simulink model "mixTest123"  (R2020a)
settings: Solver=VariableStepAuto  StartTime=0.0  StopTime=1000  FixedStep=0.05  RelTol=1e-3
InitFcn:
  | data_current
values from neighbouring files (symbols this model uses):
  a1 = rho * D^4 * alpha1    (= 0.000388302366464)    [data_current.m]    (also in main_init.m)
  a2 = -rho * D^3 * alpha2 * (1 - omega)    (= 0.0037030698432)    [data_current.m]    (also in main_init.m)
  ag = [Ax Ay Az]'    [init_modello.m]
  alpha1 = 0.0113    [data_current.m]    (also in main_init.m)
  alpha2 = -0.0091    [data_current.m]    (also in main_init.m)
  areaOfInterestCorner = [42.317744;10.915136; 0]    [init_controllo.m]    (also in missionA.m = [42.317744)
  bg = [Bx By Bz]'    [init_modello.m]
  cd_pitch = 0.7    [init_modello.m]
  cd_roll = 0.04    [init_modello.m]
  cd_x = 0.4    [init_modello.m]
  cd_y = 1    [init_modello.m]
  cd_yaw = 0.7    [init_modello.m]
  cd_z = 1    [init_modello.m]
  cg = [Cx Cy Cz]'    [init_modello.m]
  D = 0.076    [data_current.m]    (also in main_init.m)
  dead_zone_limit = 31.5    [data_current.m]    (also in main_init.m)
  dg = [Dx Dy Dz]'    [init_modello.m]
  eg = [Ex Ey Ez]'    [init_modello.m]
  fg = [Fx Fy Fz]'    [init_modello.m]
  g = 9.81    [init_modello.m]
  galleggiamento = 66.5386    [init_controllo.m]
  gg = [Gx Gy Gz]'    [init_modello.m]
  H0 = 0    [init_modello.m]
  init_position = [pointP(1),pointP(2),0.15,0,0,deg2rad(angle)]'    [appunti.m]    (also in init_modello.m = [pointP(1),pointP(2),0.15,0,0,deg2rad(alpha)]')
  init_velocity = [0 0 0 0 0 0]'    [init_modello.m]
  Ixx = 0.93304097392    [init_modello.m]
  Ixy = 0    [init_modello.m]
  Ixz = 0    [init_modello.m]
  Iyy = 25.58745481378    (= 25.5874548138)    [init_modello.m]
  Iyz = 0    [init_modello.m]
  Izz = 25.58745481378    (= 25.5874548138)    [init_modello.m]
  K_i_heave_div = 20    [init_controllo.m]
  K_i_heave_pos = 1    [init_controllo.m]
  K_i_heave_surf = 20    [init_controllo.m]
  K_i_heave_trans = 5    [init_controllo.m]
  K_i_heave_turn = 5    [init_controllo.m]
  K_i_pitch_div = 0    [init_controllo.m]
  K_i_pitch_pos = 0.1*0    (= 0)    [init_controllo.m]
  K_i_pitch_surf = 0    [init_controllo.m]
  K_i_pitch_trans = 0    [init_controllo.m]
  K_i_pitch_turn = 0    [init_controllo.m]
  K_i_roll_div = 0    [init_controllo.m]
  K_i_roll_pos = 0.1*0    (= 0)    [init_controllo.m]
  K_i_roll_surf = 1    [init_controllo.m]
  K_i_roll_trans = 0    [init_controllo.m]
  K_i_roll_turn = 0    [init_controllo.m]
  K_i_surge_div = 3    [init_controllo.m]
  K_i_surge_pos = 0.1679*30    (= 5.037)    [init_controllo.m]
  K_i_surge_surf = 3    [init_controllo.m]
  K_i_surge_trans = 0.1679*15    (= 2.5185)    [init_controllo.m]
  K_i_surge_turn = 0.1679*60    (= 10.074)    [init_controllo.m]
  K_i_sway_div = 6    [init_controllo.m]
  K_i_sway_pos = 5    [init_controllo.m]
  K_i_sway_surf = 3    [init_controllo.m]
  K_i_sway_trans = 2    [init_controllo.m]
  K_i_sway_turn = 50    [init_controllo.m]
  K_i_yaw_div = 0    [init_controllo.m]
  K_i_yaw_pos = 1    [init_controllo.m]
  K_i_yaw_surf = 0    [init_controllo.m]
  K_i_yaw_trans = 20    [init_controllo.m]
  K_i_yaw_turn = 3    [init_controllo.m]
  K_p_heave_div = 200    [init_controllo.m]
  K_p_heave_pos = 320    [init_controllo.m]
  K_p_heave_surf = 200    [init_controllo.m]
  K_p_heave_trans = 170    [init_controllo.m]
  K_p_heave_turn = 170    [init_controllo.m]
  K_p_phi_div = 0.15    [init_controllo.m]
  K_p_phi_pos = 1*0.1    (= 0.1)    [init_controllo.m]
  K_p_phi_surf = 0.15    [init_controllo.m]
  K_p_phi_trans = 0.1    [init_controllo.m]
  K_p_phi_turn = 0.1    [init_controllo.m]
  K_p_pitch_div = 50    [init_controllo.m]
  K_p_pitch_pos = 25    [init_controllo.m]
  K_p_pitch_surf = 50    [init_controllo.m]
  K_p_pitch_trans = 25    [init_controllo.m]
  K_p_pitch_turn = 25    [init_controllo.m]
  K_p_psi_div = 0.3    [init_controllo.m]
  K_p_psi_pos = 0.25    [init_controllo.m]
  K_p_psi_surf = 0.3    [init_controllo.m]
  K_p_psi_trans = 0.2    [init_controllo.m]
  K_p_roll_div = 10    [init_controllo.m]
  K_p_roll_pos = 0.1*40    (= 4)    [init_controllo.m]
  K_p_roll_surf = 10    [init_controllo.m]
  K_p_roll_trans = 0.1*40    (= 4)    [init_controllo.m]
  K_p_roll_turn = 4    [init_controllo.m]
  K_p_surge_div = 80    [init_controllo.m]
  K_p_surge_pos = 13.7782*2.5    (= 34.4455)    [init_controllo.m]
  K_p_surge_surf = 80    [init_controllo.m]
  K_p_surge_trans = 20    [init_controllo.m]
  K_p_surge_turn = 150    [init_controllo.m]
  K_p_sway_div = 100    [init_controllo.m]
  K_p_sway_pos = 90    [init_controllo.m]
  K_p_sway_surf = 80    [init_controllo.m]
  K_p_sway_trans = 80    [init_controllo.m]
  K_p_sway_turn = 200    [init_controllo.m]
  K_p_th_div = 0.3    [init_controllo.m]
  K_p_th_pos = 0.1    [init_controllo.m]
  K_p_th_surf = 0.3    [init_controllo.m]
  K_p_th_trans = 0.1    [init_controllo.m]
  K_p_th_turn = 0.1    [init_controllo.m]
  K_p_x_div = 0.12    [init_controllo.m]
  K_p_x_pos = 0.12    [init_controllo.m]
  K_p_x_surf = 0.12    [init_controllo.m]
  K_p_y_div = 0.6    [init_controllo.m]
  K_p_y_pos = 0.34    [init_controllo.m]
  K_p_y_surf = 0.1    [init_controllo.m]
  K_p_y_trans = 0.3    [init_controllo.m]
  K_p_y_turn = 0.3    [init_controllo.m]
  K_p_yaw_div = 70    [init_controllo.m]
  K_p_yaw_pos = 20    [init_controllo.m]
  K_p_yaw_surf = 70    [init_controllo.m]
  K_p_yaw_trans = 160    [init_controllo.m]
  K_p_yaw_turn = 60    [init_controllo.m]
  K_p_z_div = 0.35    [init_controllo.m]
  K_p_z_pos = 0.2    [init_controllo.m]
  K_p_z_surf = 0.35    [init_controllo.m]
  K_p_z_trans = 0.10    (= 0.1)    [init_controllo.m]
  K_p_z_turn = 0.1    [init_controllo.m]
  Kadd = 0    [init_modello.m]
  m = 100    [init_modello.m]    (also in retta.m = p2-p1)
  ... (+29 more)
undefined symbols (not defined in the file or in its folder): DiscIntNeverNeededParam
libraries: simulink x4
(part 3 of 5)

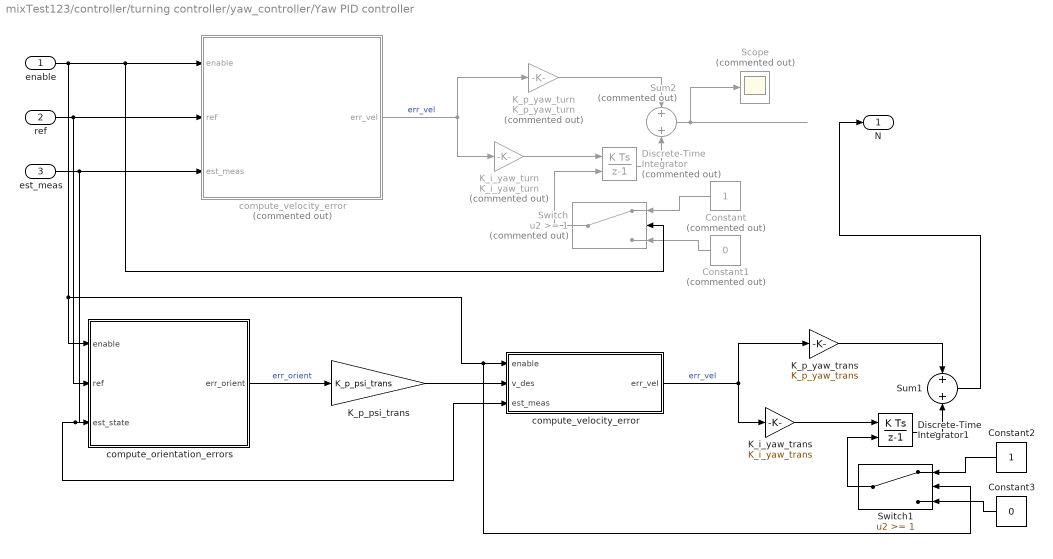
== system mixTest123/controller/turning controller/yaw_controller/Yaw PID controller ==
  enable : Inport
  ref : Inport  Port=2
  est_meas : Inport  Port=3
  " compute_velocity_error" : MATLAB Function  Commented=on  TreatAsAtomicUnit=on
  Constant : Constant  Commented=on
  Constant1 : Constant  Commented=on  Value=0
  Constant2 : Constant
  Constant3 : Constant  Value=0
  Discrete-Time Integrator : DiscreteIntegrator  Commented=on  ExternalReset=falling  SampleTime=0.1  ICPrevOutput=DiscIntNeverNeededParam  ICPrevScaledInput=DiscIntNeverNeededParam
  Discrete-Time Integrator1 : DiscreteIntegrator  ExternalReset=falling  SampleTime=0.1  ICPrevOutput=DiscIntNeverNeededParam  ICPrevScaledInput=DiscIntNeverNeededParam
  K_i_yaw_trans : Gain  Gain=K_i_yaw_trans
  K_i_yaw_turn : Gain  Commented=on  Gain=K_i_yaw_turn
  K_p_psi_trans : Gain  Gain=K_p_psi_trans
  K_p_yaw_trans : Gain  Gain=K_p_yaw_trans
  K_p_yaw_turn : Gain  Commented=on  Gain=K_p_yaw_turn
  Scope : Scope  Commented=on
  Sum1 : Sum
  Sum2 : Sum  Commented=on
  Switch : Switch  Commented=on  Threshold=1
  Switch1 : Switch  Threshold=1
  compute_orientation_errors : MATLAB Function  TreatAsAtomicUnit=on
  compute_velocity_error : MATLAB Function  TreatAsAtomicUnit=on
  N : Outport
  wires:
  Sum2/1 -> Scope/1
  " compute_velocity_error"/1(err_vel) -> K_i_yaw_turn/1, K_p_yaw_turn/1  "err_vel"
  Discrete-Time Integrator/1 -> Sum2/2
  K_p_yaw_turn/1 -> Sum2/1
  K_i_yaw_turn/1 -> Discrete-Time Integrator/1
  Switch/1 -> Discrete-Time Integrator/2
  Constant1/1 -> Switch/3
  Constant/1 -> Switch/1
  Constant3/1 -> Switch1/3
  Constant2/1 -> Switch1/1
  K_p_psi_trans/1 -> compute_velocity_error/2(v_des)
  Switch1/1 -> Discrete-Time Integrator1/2
  compute_velocity_error/1(err_vel) -> K_i_yaw_trans/1, K_p_yaw_trans/1  "err_vel"
  enable/1 -> compute_orientation_errors/1(enable), Switch1/2, compute_velocity_error/1(enable), Switch/2, " compute_velocity_error"/1(enable)
  K_i_yaw_trans/1 -> Discrete-Time Integrator1/1
  compute_orientation_errors/1(err_orient) -> K_p_psi_trans/1  "err_orient"
  est_meas/1 -> " compute_velocity_error"/3(est_meas), compute_velocity_error/3(est_meas), compute_orientation_errors/3(est_state)
  K_p_yaw_trans/1 -> Sum1/1
  ref/1 -> compute_orientation_errors/2(ref), " compute_velocity_error"/2(ref)
  Discrete-Time Integrator1/1 -> Sum1/2
  Sum1/1 -> N/1

== matlab function mixTest123/Controllo Sbaglia Depth ==
  data: u input; y output
function y = depth2alt(u)

y = zeros(12,1);

y = u;

y(3) = -u(3);

end

== stateflow chart mixTest123/Mission Supervisor/Chart ==

== matlab function mixTest123/Mission Supervisor/Trasf. in NED1 ==
  data: posArg input; pos output; areaOfInterestCorner parameter
function pos = NED2LLD(posArg,areaOfInterestCorner)
    coder.extrinsic('evalin','wgs84Ellipsoid','ned2geodetic');
    pos = zeros(1,3);
    pos1 = 0;
    pos2 = 0;
    pos3 = 0;
    [pos1, pos2, pos3] = ned2geodetic(posArg(1), posArg(2), posArg(3),areaOfInterestCorner(1), areaOfInterestCorner(2), 0,wgs84Ellipsoid);
    pos = [pos1, pos2, posArg(3)];%-posArg(3)];
end

== matlab function mixTest123/Vehicle Model/Thruster A/MATLAB Function ==
  data: n input; T output; V input; D parameter; omega parameter; a1 parameter; a2 parameter; alpha1 parameter; alpha2 parameter
function T = thrusterModel(n, V, D, omega, a1, a2, alpha1, alpha2)

Va = (1-omega) * V;     % Advancement velocity at the propeller
J0 = Va/(n*D);          % Advancement Coefficient

if J0 > -alpha1/alpha2  % Out of linearity domain (right side)
    T = 0;              % A null generated thrust is assumed
    
elseif J0 < 0           % Out of linearity domain (left side)
    T = a1*abs(n)*n;    % Bollard thrust is assumed

else                    % Within the linearity domain
    T = a1*abs(n)*n - a2*abs(n)*V;
end

== matlab function mixTest123/Vehicle Model/Thruster B/MATLAB Function ==
  data: n input; T output; V input; D parameter; omega parameter; a1 parameter; a2 parameter; alpha1 parameter; alpha2 parameter
function T = thrusterModel(n, V, D, omega, a1, a2, alpha1, alpha2)

Va = (1-omega) * V;     % Advancement velocity at the propeller
J0 = Va/(n*D);          % Advancement Coefficient

if J0 > -alpha1/alpha2  % Out of linearity domain (right side)
    T = 0;              % A null generated thrust is assumed
    
elseif J0 < 0           % Out of linearity domain (left side)
    T = a1*abs(n)*n;    % Bollard thrust is assumed

else                    % Within the linearity domain
    T = a1*abs(n)*n - a2*abs(n)*V;
end

== matlab function mixTest123/Vehicle Model/Thruster C/MATLAB Function ==
  data: n input; T output; V input; D parameter; omega parameter; a1 parameter; a2 parameter; alpha1 parameter; alpha2 parameter
function T = thrusterModel(n, V, D, omega, a1, a2, alpha1, alpha2)

Va = (1-omega) * V;     % Advancement velocity at the propeller
J0 = Va/(n*D);          % Advancement Coefficient

if J0 > -alpha1/alpha2  % Out of linearity domain (right side)
    T = 0;              % A null generated thrust is assumed
    
elseif J0 < 0           % Out of linearity domain (left side)
    T = a1*abs(n)*n;    % Bollard thrust is assumed

else                    % Within the linearity domain
    T = a1*abs(n)*n - a2*abs(n)*V;
end

== matlab function mixTest123/Vehicle Model/TAM ==
  data: Ta input; tau output double size=[6 1]; Tb input; Tc input; Td input; Te input; Tf input; Tg input; TAM parameter; eta input
function tau = fcn(Ta,Tb,Tc,Td,Te,Tf,Tg,TAM,eta)
thrust_vect = [Ta,Tb,Tc,Td,Te,Tf,Tg]';
if eta(3) >= 0
    tau = TAM*thrust_vect;
else
    tau = [0 0 0 0 0 0]';
end
end

== matlab function mixTest123/Vehicle Model/Thruster D/MATLAB Function ==
  data: n input; T output; V input; D parameter; omega parameter; a1 parameter; a2 parameter; alpha1 parameter; alpha2 parameter
function T = thrusterModel(n, V, D, omega, a1, a2, alpha1, alpha2)

Va = (1-omega) * V;     % Advancement velocity at the propeller
J0 = Va/(n*D);          % Advancement Coefficient

if J0 > -alpha1/alpha2  % Out of linearity domain (right side)
    T = 0;              % A null generated thrust is assumed
    
elseif J0 < 0           % Out of linearity domain (left side)
    T = a1*abs(n)*n;    % Bollard thrust is assumed

else                    % Within the linearity domain
    T = a1*abs(n)*n - a2*abs(n)*V;
end

== matlab function mixTest123/Vehicle Model/NED to LLDepth ==
  data: eta input double size=[6 1]; areaOfInterestCorner parameter; pos_true output double size=[3 1]; H0 parameter
function pos_true = fcn(eta,areaOfInterestCorner,H0)
coder.extrinsic('wgs84Ellipsoid');    % Reference spheroid
coder.extrinsic('ned2geodetic');
wgs84 = wgs84Ellipsoid('meter');
pos_true = zeros(3,1);
xNorth = eta(1);
yEast = eta(2);
zDown = eta(3);
LAT_AOIC = areaOfInterestCorner(1);
LON_AOIC = areaOfInterestCorner(2);
[Lat, Lon] = ned2geodetic(xNorth, yEast, zDown, LAT_AOIC, LON_AOIC, H0, wgs84,'degrees');
depth = zDown;
pos_true = [Lat, Lon, depth]';
end

== matlab function mixTest123/Vehicle Model/Coriolis computation ==
  data: nir input; C_effect output double size=[6 1]; m parameter; Ixx parameter; Iyy parameter; Izz parameter; Ixy parameter; Ixz parameter; Iyz parameter; Zadd parameter; Yadd parameter; Xadd parameter; Madd parameter; Nadd parameter; Kadd parameter
function C_effect = fcn(nir, m, Ixx, Iyy, Izz, Ixy, Ixz, Iyz, Zadd, Yadd, Xadd, Madd, Nadd, Kadd)
u = nir(1);
v = nir(2);
w = nir(3);
p = nir(4);
q = nir(5);
r = nir(6);

C11RB = zeros(3);
C12RB = m*[0 w -v;-w 0 u;v -u 0];
C21RB = -C12RB';
C22RB = [0 (-Iyz*q-Ixz*p+Izz*r) (Iyz*r+Ixy*p-Iyy*q);(Iyz*q+Ixz*p-Izz*r) 0 (-Ixz*r-Ixy*q+Ixx*p);-(Iyz*r+Ixy*p-Iyy*q) (Ixz*r+Ixy*q-Ixx*p) 0];
Crb = [C11RB C12RB;C21RB C22RB];

CA11 = zeros(3);
CA12 = [0 -Zadd*w Yadd*v;Zadd*w 0 -Xadd*u;-Yadd*v Xadd*u 0];
CA21 = -CA12';
CA22 = [0 -Nadd*r Madd*q;Nadd*r 0 -Kadd*p;-Madd*q Kadd*p 0];
Ca = [CA11 CA12;CA21 CA22];

C = Crb+Ca;
C_effect = C*nir;
end

== matlab function mixTest123/Vehicle Model/Damping computation ==
  data: nir input; D_effect output double size=[6 1]; cd_x parameter; cd_y parameter; cd_z parameter; cd_roll parameter; cd_pitch parameter; cd_yaw parameter; S_x parameter; S_y parameter; S_z parameter; S_roll parameter; S_pitch parameter; r_mz parameter; r_my parameter; r_mx parameter; S_yaw parameter; rho parameter
function D_effect = fcn(nir, cd_x, cd_y, cd_z, cd_roll, cd_pitch, cd_yaw, S_x, S_y, S_z, S_roll, S_pitch, r_mz, r_my, r_mx, S_yaw, rho)
%Calcolo matrice di Damping

vx = abs(nir(1));
vy = abs(nir(2));
vz = abs(nir(3));
wr = abs(nir(4));
wp = abs(nir(5));
wy = abs(nir(6));

D_x = -(1/2)*rho*cd_x*S_x*vx; %kg/m^3 * m^2 * m/s = kg/s (*m/s = N)
D_y = -(1/2)*rho*cd_y*S_y*vy;
D_z = -(1/2)*rho*cd_z*S_z*vz;

D_r = -(1/2)*rho*cd_roll*S_roll*((r_mx)^3)*wr; %kg/m^3 * m^2 * m^3 * 1/s = kg*m^2/s (*1/s = Nm)
D_p = -(1/2)*rho*cd_pitch*S_pitch*((r_my)^3)*wp;
D_yaw = -(1/2)*rho*cd_yaw*S_yaw*((r_mz)^3)*wy;

D = -blkdiag(D_x,D_y,D_z,D_r,D_p,D_yaw);

D_effect = D*nir;
end

== matlab function mixTest123/Vehicle Model/Gravity computation ==
  data: g_effect output double size=[6 1]; J1 input double size=[3 3]; Rb parameter; Rg parameter; W parameter; eta input; V parameter; rho parameter; g parameter
function g_effect = fcn(J1, Rb, Rg, W, eta,V, rho, g)
B = V*rho*g*[0 0 -1]'; %Forza galleggiamento in terna NED
J1_inv = inv(J1);
Fw = J1_inv*W; %Peso in terna Body
if eta(3) < -0.15
    Fb = [0,0,0]';
else
    if eta(3) <= 0.15
        B = ((eta(3)+0.15)/0.3)*B;
        Fb = J1_inv*B; %Galleggiamento in terna Body
    else
        Fb = J1_inv*B; %Galleggiamento in terna Body
    end
end
g_effect = -[Fw+Fb;cross(Rg,Fw)+cross(Rb,Fb)];
end

== matlab function mixTest123/Vehicle Model/Thruster E/MATLAB Function ==
  data: n input; T output; V input; D parameter; omega parameter; a1 parameter; a2 parameter; alpha1 parameter; alpha2 parameter
function T = thrusterModel(n, V, D, omega, a1, a2, alpha1, alpha2)

Va = (1-omega) * V;     % Advancement velocity at the propeller
J0 = Va/(n*D);          % Advancement Coefficient

if J0 > -alpha1/alpha2  % Out of linearity domain (right side)
    T = 0;              % A null generated thrust is assumed
    
elseif J0 < 0           % Out of linearity domain (left side)
    T = a1*abs(n)*n;    % Bollard thrust is assumed

else                    % Within the linearity domain
    T = a1*abs(n)*n - a2*abs(n)*V;
end

== matlab function mixTest123/Vehicle Model/Thruster F/MATLAB Function ==
  data: n input; T output; V input; D parameter; omega parameter; a1 parameter; a2 parameter; alpha1 parameter; alpha2 parameter
function T = thrusterModel(n, V, D, omega, a1, a2, alpha1, alpha2)

Va = (1-omega) * V;     % Advancement velocity at the propeller
J0 = Va/(n*D);          % Advancement Coefficient

if J0 > -alpha1/alpha2  % Out of linearity domain (right side)
    T = 0;              % A null generated thrust is assumed
    
elseif J0 < 0           % Out of linearity domain (left side)
    T = a1*abs(n)*n;    % Bollard thrust is assumed

else                    % Within the linearity domain
    T = a1*abs(n)*n - a2*abs(n)*V;
end

== matlab function mixTest123/Vehicle Model/MATLAB Function1 ==
  data: nir input double size=[6 1]; J1 input double size=[3 3]; ni_abs output double size=[6 1]; current_speed parameter double size=[3 1]
function ni_abs= fcn(nir,J1,current_speed)
J1_inv = inv(J1);
current_speed_Body = J1_inv*current_speed; %NED to Body computation
nir1 = [nir(1) nir(2) nir(3)]';
ni1_abs = nir1+current_speed_Body;
ni_abs = [ni1_abs(1) ni1_abs(2) ni1_abs(3) nir(4) nir(5) nir(6)]';
end

== matlab function mixTest123/Vehicle Model/J computation ==
  data: J output double size=[6 6]; eta input double size=[6 1]
function J  = fcn(eta)
phi = eta(4);
theta = eta(5);
psi = eta(6);
Rx = [1 0 0;0 cos(phi) sin(phi);0 -sin(phi) cos(phi)];
Ry = [cos(theta) 0 -sin(theta);0 1 0;sin(theta) 0 cos(theta)];
Rz = [cos(psi) sin(psi) 0;-sin(psi) cos(psi) 0; 0 0 1];
J1 = Rz'*Ry'*Rx';
J2_inv = [1 0 -sin(theta);0 cos(phi) (cos(theta)*sin(phi));0 -sin(phi) (cos(theta)*cos(phi))];
J2 = inv(J2_inv);
J = [J1 zeros(3);zeros(3) J2];
end

== matlab function mixTest123/Vehicle Model/MATLAB Function2 ==
  data: eta input double size=[6 1]; orient_true output
function orient_true = fcn(eta)
coder.extrinsic('wrapToPi');
orient_true = [0; 0; 0];
rr = eta(4);
r = wrapToPi(rr); %phi
pp = eta(5);
p = wrapToPi(pp); %theta
yy = eta(6);
y = wrapToPi(yy); %psi
orient_true = [r p y]';
end

== matlab function mixTest123/Vehicle Model/MATLAB Function3 ==
  data: ni_abs input double size=[6 1]; vel_true output double size=[3 1]
function vel_true = fcn(ni_abs)
vx = ni_abs(1);
vy = ni_abs(2);
vz = ni_abs(3);
vel_true = [vx,vy,vz]';
end

== matlab function mixTest123/Vehicle Model/MATLAB Function4 ==
  data: ni_abs input double size=[6 1]; w_true output double size=[3 1]
function w_true = fcn(ni_abs)
w_x = ni_abs(4);
w_y = ni_abs(5);
w_z = ni_abs(6);
w_true = [w_x,w_y,w_z]';
end

== matlab function mixTest123/Vehicle Model/Thruster G/MATLAB Function ==
  data: n input; T output; V input; D parameter; omega parameter; a1 parameter; a2 parameter; alpha1 parameter; alpha2 parameter
function T = thrusterModel(n, V, D, omega, a1, a2, alpha1, alpha2)

Va = (1-omega) * V;     % Advancement velocity at the propeller
J0 = Va/(n*D);          % Advancement Coefficient

if J0 > -alpha1/alpha2  % Out of linearity domain (right side)
    T = 0;              % A null generated thrust is assumed
    
elseif J0 < 0           % Out of linearity domain (left side)
    T = a1*abs(n)*n;    % Bollard thrust is assumed

else                    % Within the linearity domain
    T = a1*abs(n)*n - a2*abs(n)*V;
end

== matlab function mixTest123/Vehicle Model/Velocità_ai_thruster ==
  data: nir input double size=[6 1]; Va_rel output; Vb_rel output; Vc_rel output; Vd_rel output; Ve_rel output; Vf_rel output; Vg_rel output; orA parameter; orB parameter; orC parameter; orD parameter; orE parameter; orF parameter; orG parameter; ag parameter; bg parameter; cg parameter; dg parameter; eg parameter; fg parameter; gg parameter
function [Va_rel,Vb_rel,Vc_rel,Vd_rel,Ve_rel,Vf_rel,Vg_rel] = fcn(nir, orA, orB, orC, orD, orE, orF, orG, ag, bg, cg, dg, eg, fg, gg)
nir1 = [nir(1) nir(2) nir(3)]';
nir2 = [nir(4) nir(5) nir(6)]';
%Vettori orientazione thrusterX denominati orX  disponibili nel file init
%Vettori posizione thrusterX denominati xg disponibili nel file init
Va_rel = orA*(nir1 + cross(nir2,ag));
Vb_rel = orB*(nir1 + cross(nir2,bg));
Vc_rel = orC*(nir1 + cross(nir2,cg));
Vd_rel = orD*(nir1 + cross(nir2,dg));
Ve_rel = orE*(nir1 + cross(nir2,eg));
Vf_rel = orF*(nir1 + cross(nir2,fg));
Vg_rel = orG*(nir1 + cross(nir2,gg));
[Va_rel,Vb_rel,Vc_rel,Vd_rel,Ve_rel,Vf_rel,Vg_rel];
end

== matlab function mixTest123/Vehicle Model/J1 computation ==
  data: eta input; J1 output
function J1 = fcn(eta)
phi = eta(4);
theta = eta(5);
psi = eta(6);
Rx = [1 0 0;0 cos(phi) sin(phi);0 -sin(phi) cos(phi)];
Ry = [cos(theta) 0 -sin(theta);0 1 0;sin(theta) 0 cos(theta)];
Rz = [cos(psi) sin(psi) 0;-sin(psi) cos(psi) 0; 0 0 1];
J1 = Rz'*Ry'*Rx';
end

== matlab function mixTest123/Vehicle Model/ni_dot computation ==
  data: M_times_nir_dot input double size=[6 1]; nir_dot output double size=[6 1]; M_inv parameter
function nir_dot = fcn(M_times_nir_dot, M_inv)
nir_dot = M_inv * M_times_nir_dot;
end

== matlab function mixTest123/Vehicle Model/ni_to_eta_dot ==
  data: J input; ni_abs input; eta_dot output
function eta_dot = fcn(J,ni_abs)
eta_dot = J*ni_abs;
end

== stateflow chart mixTest123/Mission Supervisor1/Chart ==

== matlab function mixTest123/Mission Supervisor1/Trasf. in NED ==
  data: posArg input; pos output; areaOfInterestCorner parameter
function pos = LLD2NED(posArg,areaOfInterestCorner)
    coder.extrinsic('evalin','wgs84Ellipsoid','geodetic2ned');
    pos = zeros(1,3);
    pos1 = 0;
    pos2 = 0;
    pos3 = 0;
    [pos1, pos2, pos3] = geodetic2ned(posArg(1), posArg(2), posArg(3),areaOfInterestCorner(1), areaOfInterestCorner(2), 0,wgs84Ellipsoid);
    pos = [pos1, pos2, posArg(3)];
end

== stateflow chart mixTest123/Mission Supervisor1/State Management ==
  state Movements [parallel]
    settings: executionOrder=1
    state End [function]
    state positioning
      entry:
      current_state(1:5) = [1 0 0 0 0];
      orBene = 0;
      velNull = 0;
      fromFirstPos = 0;
      during:
      if ~missionEnd %missione appena iniziata
      if ~checkOr([0,0,orDes],orient,errOrPos) && ~orBene
      pos_ref = pointP;
      orient_ref = [0,0,orDes];
      vel_ref = [0,0,0,0,0,0];
      else%orientato bene, dentro o fuori sfera
      orBene=1;
      pos_ref = pointA;
      orient_ref = [0,0,orDes];
      vel_ref = velPos;
      end
      else %missione completata con successo
      pos_ref = pointP;
      orient_ref = [0,0, orDesRit];
      vel_ref = velPos;
      end
    state diving
      entry:
      current_state(1:5) = [0 1 0 0 0];
      velNull = 0;
      during:
      if ~(checkPos(pointA,pos, errSphere) && checkOr([0,0,orDes],orient,errOrPos) ...
      && checkVel(zeros(1,6),[vel(1),vel(2),vel(3),0,0,0],errVelDiv)) && ~velNull
      pos_ref = pointA;
      orient_ref = [0,0,orDes];
      vel_ref = zeros(1,6);
      else
      velNull = 1;
      pos_ref = [pointA(1),pointA(2), averageDepth - altitude];
      orient_ref = orientA;
      if (pos_ref(3) - pos(3) > endDiv)
      vel_ref = velSub;
      else
      vel_ref = velRidSub;
      end
      end
    state surfacing
      entry:
      current_state(1:5) = [0 0 0 0 1];
      velNull = 0;
      during:
      if wall || current_state(8)
      pos_ref = [pos(1), pos(2), 0.15];
      else
      if ~checkVel(zeros(1,6),[vel(1),vel(2),vel(3),0,0,0],errVelSurf) && ~velNull
      pos_ref = trWP(nWPTran,:,nTran);
      orient_ref = [0,0,orDesRit];
      vel_ref = zeros(1,6);
      else
      velNull = 1;
      ptSup = trWP(nWPTran,:,nTran);
      pos_ref = [ptSup(1),ptSup(2),0.15];
      orient_ref = [0,0,orDesRit];
      vel_ref = velSurf;
      end
      end
    state transect
      entry:
      current_state(1:5) = [0 0 1 0 0];
      ptx = trWP(wpTR,:,page);
      pos_ref = [ptx(1),ptx(2),pos(3)-(altitude-FLS_down)];
      if mod(page,2) == 0
      orient_ref = orPari;
      else
      orient_ref = orDispari;
      end
      vel_ref = velTran;
      state Disaligned
        (default) -> (junction 490)
        (junction 490) -> (junction 207) : {sizeEmerg = size(wpEmerg);}
        (junction 207) -> (junction 674) [order 1] : [~all(sizeEmerg)]
        (junction 674) -> (junction 681) [order 2] : {wpTR = nWPTran;}
        (junction 207) -> (junction 210) [order 2]
        (junction 674) -> (junction 681) [order 1] : [wpTR + 2 <= nWPTran]
            | {wpTR = wpTR+2;}
        (junction 681) -> (junction 210) : {wpEmerg = currentSwingWaypoints(trWP(wpTR,:,page),pos,distEmerg);}
        (junction 210) -> (junction 396) : {ptx = wpEmerg(idxEmerg,1:3);
            | pos_ref = [ptx(1),ptx(2),pos(3)-(altitude-FLS_down)];
            | vel_ref = vEmergTran;}
        (junction 396) -> (junction 225) [order 1] : [mod(page,2) == 0]
            | {orient_ref = orPari;}
        (junction 396) -> (junction 225) [order 2] : {orient_ref =orDispari;}
        (junction 225) -> (junction 259) [order 2]
        (junction 225) -> (junction 213) [order 1] : [checkPos(pos,pos_ref,errPosWPTrans) &&...
            | checkOr(orient,orient_ref,errOrWPTrans)]
        (junction 213) -> (junction 215) [order 1] : [idxEmerg == size(wpEmerg,1)]
            | {idxEmerg = 1; current_state(6) = 0;}
        (junction 213) -> (junction 215) [order 2] : {idxEmerg = idxEmerg + 1;}
      state Aligned
        (default) -> (junction 203)
        (junction 203) -> (junction 754) [order 2] : {error=errPosTransLast;}
        (junction 203) -> (junction 754) [order 1] : [wpTR<=nWPTran-2]
            | {error=errPosTrans;}
        (junction 754) -> (junction 219) [order 2]
        (junction 754) -> (junction 663) [order 1] : [checkPos(pos_ref,pos,error) && ...
            | checkOr(orient_ref,orient,errOrTrans)]
        (junction 663) -> (junction 219) : [wpTR+1 <= nWPTran]
            | {wpTR = wpTR + 1;} %indica WP successivo
        (junction 219) -> (junction 393) : {wpEmerg =  [];
            | ptx = trWP(wpTR,:,page);
            | pos_ref = [ptx(1),ptx(2),pos(3)-(altitude-FLS_down)];}
        (junction 393) -> (junction 222) [order 1] : [mod(page,2) == 0]
            | {orient_ref = orPari;}
        (junction 393) -> (junction 222) [order 2] : {orient_ref = orDispari;}
        (junction 222) -> (junction 227) [order 1] : [wpTR > nWPTran - 2]
            | {vel_ref = velRid;}
        (junction 222) -> (junction 227) [order 2] : {vel_ref = velTran;}
      Aligned -> Aligned [order 2]
      Disaligned -> Disaligned [order 2]
      (default) -> Aligned
      Disaligned -> Aligned [order 1] : [~current_state(6)]
      Aligned -> Disaligned [order 1] : [current_state(6)]
    state turn
      entry:
      current_state(1:5) = [0 0 0 1 0];
      state ReferencePoints
        (default) -> (junction 728)
        (junction 728) -> (junction 736) [order 2] : {pos_ref = turnWP(nWPTurn,:,page);
            | orient_ref = deg2rad(turnRef(nWPTurn,:,page));}
        (junction 728) -> (junction 733) [order 1] : [time+1<=nWPTurn]
            | {pos_ref = turnWP(time+1,:,page);
            | orient_ref = deg2rad(turnRef(time+1,:,page));}
        (junction 736) -> (junction 733)
        (junction 733) -> (junction 738) [order 1] : [mod(page,2) == 0]
            | {vel_ref = [0.2 0 0 0 0 -rot*0.2/(lineSpaceBetweenTransects/2)];}
        (junction 733) -> (junction 731) [order 2] : {vel_ref = [0.2 0 0 0 0 rot*0.2/(lineSpaceBetweenTransects/2)];}
      ReferencePoints -> ReferencePoints
      (default) -> ReferencePoints
    (default) -> positioning : {missionEnd = 0;}
    positioning -> positioning [order 1] : [missionEnd && checkPos(pointP,pos,errPosPos/2)]
        | {End();}
    positioning -> diving [order 2] : [checkPos(pointA,pos,errPosPos) && checkOr([0,0,orDes],orient,errOrPos)]
    positioning -> surfacing [order 3] : [wall || current_state(8)]
        | {fromFirstPos = 1;}
    surfacing -> positioning : [checkPos3([ptSup(1),ptSup(2),0.15],pos,errPosSurf) && ...
        | checkOr([0,0,orDesRit],orient,errOrSurf) && checkVel(zeros(1,6),vel,errVelSurf)...
        | && ~fromFirstPos]
        | {missionEnd = 1;}
    diving -> surfacing [order 2] : [wall || current_state(8)]
    diving -> transect [order 1] : [checkPos3([pointA(1),pointA(2), pos(3)-(altitude-FLS_down)],pos,errPosDiv) ...
        | && checkOr(orientA,orient,errOrDiv)]
    transect -> surfacing [order 1] : [wall || current_state(8)]
    turn -> surfacing [order 2] : [wall || current_state(8)]
    transect -> surfacing [order 2] : [(checkPos(trWP(nWPTran,:,nTran),pos, errPosTrans) &&...
        | checkOr(orient_ref,orient,errOrTrans))]
    turn -> transect [order 1] : [time+1 == nWPTurn]
        | {page = page + 1; wpTR = 1;}
    transect -> turn [order 3] : [checkPos(trWP(nWPTran,:,page),pos, errPosTransLast) && checkOr(orient_ref,orient,errOrTrans)]
        | {wpTU=1;}
  state Issues_management [parallel]
    entry:
    points=[];
    profs=[];
    settings: executionOrder=2
    state Free
      entry:
      current_state(6:8) = 0;
      during:
      if current_state(1) || current_state(5)
      pos_ref(3) = 0.15;
      else
      if abs(altitude - FLS_down)>=minGap
      pos_ref(3)= pos(3) - (altitude - FLS_down);
      else
      pos_ref(3) = pos(3);
      end
      end
    state Issue_found
      state obstacle %parete/ostacoli [parallel]
        during:
        distFront = FLS_front*cos(deg2rad(theta_f));
        distDown = FLS_front*sin(deg2rad(theta_f));
        nedFLS = fix2LocalNED(orient(1),orient(2),orient(3))'*[distFront;0;distDown];
        pointProf = pos(3) - (altitude-FLS_down) - (FLS_down-nedFLS(3));
        pointApp = calcPoint(pos,orient,nedFLS(1));
        nedAxis = (fix2LocalNED(orient(1),orient(2),orient(3))'*[semix; semiy; semiz])';
        settings: executionOrder=3
        (default) -> (junction 563)
        (junction 563) -> (junction 575) [order 2] : [~all(size(points))]
            | %{current_state(7) = 0;}
        (junction 563) -> (junction 565) [order 1] : [all(size(points))]
            | {distObsVeh = distance(pos+nedAxis,points(1,:));
            | punto = points(1,:);}
        (junction 565) -> (junction 789) [order 2] : [distObsVeh>(abs(pos(3)-profs(1))...
            | /maxRatio + safeMargin)]
        (junction 565) -> (junction 567) [order 1] : [distObsVeh<=(abs(pos(3)-profs(1))/maxRatio + safeMargin)]
            | {pos_ref(3) = profs(1);}
        (junction 575) -> (junction 573)
        (junction 567) -> (junction 791)
        (junction 789) -> (junction 791)
        (junction 791) -> (junction 573) [order 2]
        (junction 791) -> (junction 573) [order 1] : [checkPos([punto(1),punto(2),profs(1)],pos,errPosPos)]
            | {points  = points(2:end,:);}
        (junction 573) -> (junction 578) [order 1] : [(pos(3) - pointProf)/(distFront+nedAxis(1)) > maxRatio]
            | {current_state(7) = 1;wall = 1;}
        (junction 573) -> (junction 605) [order 3]
        (junction 573) -> (junction 580) [order 2] : [(pos(3) - pointProf)/(distFront+nedAxis(1)) <= maxRatio]
        (junction 580) -> (junction 582) [order 1] : [all(size(points))]
            | {distObs = distance(points(end,:),pointApp);}
        (junction 580) -> (junction 794) [order 2] : [~all(size(points))]
        (junction 794) -> (junction 796) [order 2]
        (junction 794) -> (junction 586) [order 1] : [pos(3)-pointProf>=minGap]
            | {distObsVeh=distance(pos,pointApp)}
        (junction 582) -> (junction 785) [order 2]
        (junction 582) -> (junction 584) [order 1] : [abs(profs(end)-pointProf)>=minGap]
        (junction 586) -> (junction 787) [order 2]
        (junction 586) -> (junction 588) [order 1] : [distObsVeh>=minDist+nedAxis(1)]
            | {points = cat(1,points,pointApp);}
        (junction 584) -> (junction 590) [order 1] : [distObs < minDist || (profs(end)-pointProf)/distObs > maxRatio]
            | {points = points(1:end-1,:);}
        (junction 584) -> (junction 592) [order 2]
        (junction 590) -> (junction 592)
        (junction 592) -> (junction 595) : {points=cat(1,points,pointApp);}
      state warning %disallineamento [parallel]
        during:
        if current_state(3)
        disalignOP;
        end
        if abs(altitude - FLS_down)>=minGap
        pos_ref(3)= pos(3) - (altitude - FLS_down);
        else
        pos_ref(3) = pos(3);
        end
        settings: executionOrder=1
      state abort %danni strutturali [parallel]
        entry:
        inactivity = 1;
        during:
        checkFailure;
        settings: executionOrder=2
      state disalignOP [function]
        (default) -> (junction 696)
        (junction 696) -> (junction 700) [order 1] : [current_state(3) && wpTR >=2 &&...
            | retta(pos,trWP(1,:,page),trWP(nWPTran,:,page))>=offset]
            | {current_state(6) = 1;}
        (junction 696) -> (junction 747) [order 2] : [current_state(3) && wpTR>nWPTran-2 ...
            | && retta(pos,trWP(1,:,page),trWP(nWPTran,:,page))>=offsetLast]
            | {current_state(6) = 1;}
        (junction 696) -> (junction 780) [order 3]
      state checkFailure [function]
        (default) -> (junction 108)
        (junction 109) -> (junction 114) : [mod(inactivity,1000) == 0]
            | {current_state(8) = 1;}
        (junction 108) -> (junction 109) : [vel(1:3) == [0 0 0]]
            | {inactivity = inactivity + 1;}
    state rit = check [function]
      note: (abs(pos(2)-pos_ref(2))>=offset || abs(pos(1)-pos_ref(1))>=offset))
      (default) -> (junction 690)
      (junction 690) -> (junction 122) : {cur_dir = ned2Traj(rad2deg(orient(3)))'*[1;0;0];
          | err_dir = pos(2) - cur_dir(2);}
      (junction 122) -> (junction 479) [order 2] : {rit = 0;}
      (junction 122) -> (junction 124) [order 1] : [(current_state(3) && abs(err_dir)>=offset) || all(size(points)) ]
          | {rit = 1;}%|| checkWall || checkFailure
    (default) -> Free
    Free -> Issue_found : [check]
    Issue_found -> Free : [~check]
  data: puntoDes function_input; puntoCorr function_input; dist function_input; M function_output; ang constant double =angle; vRef function_input; vAct function_input; vErr function_input; okVel function_output; oRef function_input; oAct function_input; oErr function_input; okOr function_output; pRef function_input; pAct function_input; pErr function_input; okPos function_output; pRef function_input; pAct function_input; pErr function_input; okPos function_output; p1 function_input; p2 function_input; valDist function_output; distPR function_output; position function_input; p1 function_input; p2 function_input; phi function_input; theta function_input; rotation function_output; psi function_input; ang function_input; rotation function_output; p function_input; o function_input; pt function_output; d function_input; pRef function_input; oRef function_input; vRef function_input; pAct function_input; oAct function_input; vAct function_input; pErr function_input; oErr function_input; vErr function_input; placed function_output; vRef function_input; vAct function_input; vErr function_input; okVel function_output; oRef function_input; oAct function_input; oErr function_input; okOr function_output; pRef function_input; pAct function_input; pErr function_input; okPos function_output; pRef function_input; pAct function_input; pErr function_input; okPos function_output; rit function_output; current_state output size=[1, 8] =[0 0 0 0 0 0 0 0]; pos_ref output =pointP; orient_ref output size=[1 3] =[0 0 deg2rad(angle)]; pos input; orient input; vel input; FLS_front input; FLS_down input; time input; vel_ref output =[0 0 0 0 0 0]; orientA parameter; velPos parameter; velSub parameter; velSurf parameter; velTran parameter; wpEmerg local size=[200 3] =zeros(200,3); altitude parameter; averageDepth parameter; nTran parameter; nWPTran parameter; nWPTurn parameter; pointP parameter; trWP parameter; turnWP parameter; velRid parameter; idxEmerg local =1; missionEnd local =0; endDiv parameter; turnRef parameter; velRidSub parameter; errOrDiv parameter; errOrSurf parameter; errOrTrans parameter; errOrWPTrans parameter; errPosDiv parameter; errPosSurf parameter; errPosTrans parameter; errPosWPTrans parameter; errVelDiv parameter; errVelSurf parameter; inactivity local =1; errOrPos parameter; errPosPos parameter; errVelPos parameter; vEmergTran parameter; angle parameter; offset parameter; sizeEmerg local size=[1,2] =[0 0]; distEmerg parameter; pointA parameter; wpTR local =1; wpTU local =1; page local =1; maxRatio parameter; minDist parameter; minGap parameter; profs local size=[1 20] =zeros(1,20); semix parameter; semiy parameter double; semiz parameter; theta_f parameter; distObsVeh local size=1 =0; distDown local size=1 =0; distFront local size=1 =0; nedAxis local size=[1,3] =zeros(1,3); nedFLS local; pointApp local size=[1,2] =zeros(1,2); pointProf local size=[1 1] =0; points local size=[20 2] =zeros(20,2); distObs local size=1 =0; safeMargin parameter; orDes parameter; orBene local; velNull local; errSphere parameter; ptx local =[0 0 0]; lineSpaceBetweenTransects parameter; ptSup local size=[1 3] =zeros(1,3); orDesRit parameter; orDispari parameter; orPari parameter; fromFirstPos local; wall local =0; cur_dir local; err_dir local; rot parameter; errPosTransLast parameter; error local; offsetLast parameter; cur_pos local; punto local size=[1 3]
  function M = currentSwingWaypoints(puntoDes,puntoCorr,dist):
    | function M = currentSwingWaypoints(puntoDes,puntoCorr,dist)
    | %Generazione di waypoint aggiuntivi supponendo di conoscere il punto finale
    | % desiderato sul transetto
    | %
    | %   -puntoDes: punto desiderato sulla traiettoria rettilinea; 1x3 [m m m]
    | %   -puntoCorr: punto stimato di posizione corrente; 1x3 [m m m]
    | %   -dist: distanza tra waypoint; [m]
    | 
    | %     %lunghezza segmento
    | %     lunghezza= sqrt((puntoCorr(1) - puntoDes(1))^2 +(puntoCorr(2)-puntoDes(2))^2);% + (puntoCorr(3) - puntoDes(3))^2); 
    | %     
    | %     p = floor(lunghezza/dist); %numero waypoint
    | 
    |     distN = puntoCorr(1) - puntoDes(1); %distanza su N tra punto iniziale e finale
    |     distE = puntoCorr(2) - puntoDes(2); %distanza su E tra punto iniziale e finale
    | %     distD = puntoCorr(3) - puntoDes(3); %distanza su D tra punto iniziale e finale
    | 
    |     p = floor(abs(distE)/dist);
    |     
    |     deltaE = distE/p; %distanza tra waypoints su East
    |     deltaN = distN/p; %distanza tra waypoints su North
    | %     deltaD = distD/p; %distanza tra waypoints su Down
    |    
    |     matrix = zeros(p-1,3);
    |    
    |     for i = 1:p-1 %possiamo fermarci a p-1 perché waypoint su traiettoria già fornito
    |         waypoint = puntoCorr - i * [deltaN deltaE 0];
    |         waypoint(3) = puntoDes(3);%deltaD];
    |         matrix(i,:) = waypoint;%matrix = cat(1, matrix, waypoint);
    |     end
    |     %matrix = cat(2, matrix, puntoDes);
    |     M = matrix;   
    |    
    | end
  function okVel = checkVel(vRef,vAct,vErr):
    | function okVel = checkVel(vRef,vAct,vErr)
    | %Funzione che controlla che il posizionamento sull'angolo dell'area interessata
    | % sia effettivamente avvenuto, per segnalare l'inizio della fase di
    | % immersione
    | %   -vRef: velocità desiderata; 1x6 [m/s m/s m/s rad/s rad/s rad/s]
    | %   -vAct: velocità corrente; 1x3 [m/s m/s m/s rad/s rad/s rad/s]
    | %   -vErr: errore accettabile in velocità; 1x3 [m/s m/s m/s rad/s rad/s rad/s]
    | 
    |     okVel = all(abs(vRef - vAct) <= vErr); %check su velocità
    | end
  function okOr = checkOr(oRef,oAct,oErr):
    | function okOr = checkOr(oRef,oAct,oErr)
    | %Funzione che controlla che il posizionamento sull'angolo dell'area interessata
    | % sia effettivamente avvenuto, per segnalare l'inizio della fase di
    | % immersione
    | %   -oRef: orientazione desiderata; 1x3 [° ° °]
    | %   -oAct: orientazione corrente, stimata dalla navigazione; 1x3 [° ° °]
    | %   -oErr: errore accettabile in orientamento; 1x3 [° ° °]
    | 
    |     okOr = all(abs(oRef - oAct) <= oErr); %check su orientazione
    | end
  function okPos = checkPos(pRef,pAct,pErr):
    | function okPos = checkPos(pRef,pAct,pErr)
    | %Funzione che controlla che il posizionamento sull'angolo dell'area interessata
    | % sia effettivamente avvenuto, per segnalare l'inizio della fase di
    | % immersione
    | %   -pRef: punto di arrivo desiderato; 1x3 [m m m]
    | %   -pAct: posizione corrente, stimata dalla navigazione; 1x3 [m m m]
    | %   -pErr: errore accettabile in posizione; 1x3 [m m m]
    | 
    |     okPos = all(abs(pRef(1:2) - pAct(1:2))  <= pErr(1:2)); %check su posizione
    | end
  function okPos = checkPos3(pRef,pAct,pErr):
    | function okPos = checkPos3(pRef,pAct,pErr)
    | %Funzione che controlla che il posizionamento sull'angolo dell'area interessata
    | % sia effettivamente avvenuto, per segnalare l'inizio della fase di
    | % immersione
    | %   -pRef: punto di arrivo desiderato; 1x3 [m m m]
    | %   -pAct: posizione corrente, stimata dalla navigazione; 1x3 [m m m]
    | %   -pErr: errore accettabile in posizione; 1x3 [m m m]
    | 
    |     okPos = all(abs(pRef - pAct)  <= pErr); %check su posizione
    | end
  function valDist = distance(p1,p2):
    | function valDist = distance(p1,p2)
    |  %p1,p2 considerati di due dimensioni
    |     valDist = sqrt((p1(1)-p2(1))^2 + (p1(2)-p2(2))^2);
    | end
  function distPR = retta(position,p1,p2):
    | function distPR = retta(position,p1,p2)
    | %Funzione che ritorna la distanza tra un punto e una retta costruita a
    | % partire da due suoi punti 
    |     m = p2-p1;
    |     coeff=m(2)/m(1);
    |     distPR = abs(position(2)-(coeff*(position(1)-p1(1))+p1(2)))/sqrt(1+coeff^2);
    |     %y-y1 = m*(x-x1) -> y = m*(x-x1)+y1
    | end
  function rotation = fix2LocalNED(phi, theta, psi):
    | function rotation = fix2LocalNED(phi, theta, psi)
    | %Matrice di rotazione generica per una rotazione RPY, da sdr fisso a sdr
    | %ruotato
    | %   -phi: angolo su asse x
    | %   -theta: angolo su asse y
    | %   -psi: angolo su asse z
    | 
    |     phirad = deg2rad(phi);
    |     cr = cos(phirad);
    |     sr = sin(phirad);
    | 
    |     thetarad = deg2rad(theta);
    |     cp = cos(thetarad);
    |     sp = sin(thetarad);
    | 
    |     psirad = deg2rad(psi);
    |     cy = cos(psirad);
    |     sy = sin(psirad);
    | 
    |     rotx = [[1 0 0];
    |             [0 cr sr];
    |             [0 -sr cr]];
    | 
    |     roty = [[cp 0 -sp];
    |             [0 1 0];
    |             [sp 0 cp]];
    | 
    |     rotz = [[cy sy 0];
    |             [-sy cy 0];
    |             [0 0 1]];
    | 
    |     rotation = rotx*roty*rotz;
    | 
    | end
  function rotation = ned2Traj(ang):
    | function rotation = ned2Traj(ang)
    | %Rotation matrix describing the transformation from the local reference
    | %system onto the trajectory to the general NED reference system,
    | %considering a simple yaw rotation
    | %
    | %   -ang: yaw angle; [°]
    | 
    |         a = deg2rad(ang);
    |         rotation = [cos(a) sin(a) 0; 
    |                -sin(a) cos(a) 0;
    |                  0 0 1];
    | end
  function pt = calcPoint(p,o,d):
    | function pt = calcPoint(p,o,d)
    |     nedDist = fix2LocalNED(o(1),o(2),o(3))'*[d; 0; 0];
    |     pt = [p(1) p(2)] + [nedDist(1) nedDist(2)];
    |     
    | end
  function placed = checkRif(pRef, oRef, vRef, pAct, oAct, vAct, pErr, oErr, vErr):
    | function placed = checkRif(pRef, oRef, vRef, pAct, oAct, vAct, pErr, oErr, vErr)
    | %Funzione che controlla che il posizionamento sull'angolo dell'area interessata
    | % sia effettivamente avvenuto, per segnalare l'inizio della fase di
    | % immersione
    | %   -pRef: punto di arrivo desiderato; 1x3 [m m m]
    | %   -oRef: orientazione desiderata; 1x3 [° ° °]
    | %   -vRef: velocità desiderata; 1x6 [m/s m/s m/s rad/s rad/s rad/s]
    | %   -pAct: posizione corrente, stimata dalla navigazione; 1x3 [m m m]
    | %   -oAct: orientazione corrente, stimata dalla navigazione; 1x3 [° ° °]
    | %   -vAct: velocità corrente; 1x3 [m/s m/s m/s rad/s rad/s rad/s]
    | %   -pErr: errore accettabile in posizione; 1x3 [m m m]
    | %   -oErr: errore accettabile in orientamento; 1x3 [° ° °]
    | %   -vErr: errore accettabile in velocità; 1x3 [m/s m/s m/s rad/s rad/s rad/s]
    | 
    |     p = abs(pRef - pAct)  <= pErr; %check su posizione
    |     o = abs(oRef - oAct) <= oErr; %check su orientazione
    |     v = abs(vRef - vAct) <= vErr; %check su velocità
    |         
    |     placed = all(p) && all(o) && all(v);
    | 
    | end
  function okVel = checkVel(vRef,vAct,vErr):
    | function okVel = checkVel(vRef,vAct,vErr)
    | %Funzione che controlla che il posizionamento sull'angolo dell'area interessata
    | % sia effettivamente avvenuto, per segnalare l'inizio della fase di
    | % immersione
    | %   -vRef: velocità desiderata; 1x6 [m/s m/s m/s rad/s rad/s rad/s]
    | %   -vAct: velocità corrente; 1x3 [m/s m/s m/s rad/s rad/s rad/s]
    | %   -vErr: errore accettabile in velocità; 1x3 [m/s m/s m/s rad/s rad/s rad/s]
    | 
    |     okVel = all(abs(vRef - vAct) <= vErr); %check su velocità
    | end
  function okOr = checkOr(oRef,oAct,oErr):
    | function okOr = checkOr(oRef,oAct,oErr)
    | %Funzione che controlla che il posizionamento sull'angolo dell'area interessata
    | % sia effettivamente avvenuto, per segnalare l'inizio della fase di
    | % immersione
    | %   -oRef: orientazione desiderata; 1x3 [° ° °]
    | %   -oAct: orientazione corrente, stimata dalla navigazione; 1x3 [° ° °]
    | %   -oErr: errore accettabile in orientamento; 1x3 [° ° °]
    | 
    |     okOr = all(abs(oRef - oAct) <= oErr); %check su orientazione
    | end
  function okPos = checkPos(pRef,pAct,pErr):
    | function okPos = checkPos(pRef,pAct,pErr)
    | %Funzione che controlla che il posizionamento sull'angolo dell'area interessata
    | % sia effettivamente avvenuto, per segnalare l'inizio della fase di
    | % immersione
    | %   -pRef: punto di arrivo desiderato; 1x3 [m m m]
    | %   -pAct: posizione corrente, stimata dalla navigazione; 1x3 [m m m]
    | %   -pErr: errore accettabile in posizione; 1x3 [m m m]
    | 
    |     okPos = all(abs(pRef(1:2) - pAct(1:2))  <= pErr(1:2)); %check su posizione
    | end
  function okPos = checkPos3(pRef,pAct,pErr):
    | function okPos = checkPos3(pRef,pAct,pErr)
    | %Funzione che controlla che il posizionamento sull'angolo dell'area interessata
    | % sia effettivamente avvenuto, per segnalare l'inizio della fase di
    | % immersione
    | %   -pRef: punto di arrivo desiderato; 1x3 [m m m]
    | %   -pAct: posizione corrente, stimata dalla navigazione; 1x3 [m m m]
    | %   -pErr: errore accettabile in posizione; 1x3 [m m m]
    | 
    |     okPos = all(abs(pRef - pAct)  <= pErr); %check su posizione
    | end

== matlab function mixTest123/Mission Supervisor1/Trasf. in NED1 ==
  data: posArg input; pos output; areaOfInterestCorner parameter
function pos = NED2LLD(posArg,areaOfInterestCorner)
    coder.extrinsic('evalin','wgs84Ellipsoid','ned2geodetic');
    pos = zeros(1,3);
    pos1 = 0;
    pos2 = 0;
    pos3 = 0;
    [pos1, pos2, pos3] = ned2geodetic(posArg(1), posArg(2), posArg(3),areaOfInterestCorner(1), areaOfInterestCorner(2), 0,wgs84Ellipsoid);
    pos = [pos1, pos2, posArg(3)];%-posArg(3)];
end

== matlab function mixTest123/controller/abort mission/abort mission ==
  data: enable input; abort output size=[6 1]; ref input; est_meas input
function abort = fcn(enable, ref, est_meas)
tau = zeros(6,1);
abort = zeros(6,1);
if enable == 1
    abort = tau;
else
    abort = tau;
end
end

== matlab function mixTest123/controller/compute n_des ==
  settings: updateMethod=DISCRETE  sampleTime=0.1
  data: enable input size=6; n_des output size=[7 1]; tau_pos input size=6; tau_div input size=6; tau_trans input size=6; tau_turn input size=6; tau_surf input size=6; abort input size=6
function n_des = fcn(enable, tau_pos, tau_div, tau_trans, tau_turn, tau_surf, abort)
j = 0;
tau = zeros(6,1);
for i=1:1:length(enable)
    if enable(i) == 1
        j = i;
    end
end
if j == 1
    tau = tau_pos;
end
if j == 2
    tau = tau_div;
end
if j == 3
    tau = tau_trans;
end
if j == 4
    tau = tau_turn;
end
if j == 5
    tau = tau_surf;
end
if j == 6
    tau = abort;
end
% Definisco la matrice di allocazione ai trust B
p_1 = [0.6  0.15 0.005]';
p_2 = [0.6 -0.15 0.005]';
p_3 = [0  0.2 0]';
p_4 = [0 -0.2 0]';
p_5 = [-1.2  0  0.005]';
p_6 = [-0.9  0  0]';
p_7 = [ 0.9  0  0]';

t_1 = [0 0 1]';
t_2 = [0 0 1]';
t_3 = [1 0 0]';
t_4 = [1 0 0]';
t_5 = [0 0 1]';
t_6 = [0 1 0]';
t_7 = [0 1 0]';

B_1 = [t_1;cross(p_1,t_1)];
B_2 = [t_2;cross(p_2,t_2)];
B_3 = [t_3;cross(p_3,t_3)];
B_4 = [t_4;cross(p_4,t_4)];
B_5 = [t_5;cross(p_5,t_5)];
B_6 = [t_6;cross(p_6,t_6)];
B_7 = [t_7;cross(p_7,t_7)];

B = [B_1 B_2 B_3 B_4 B_5 B_6 B_7];
B_pinv = pinv(B);

% Forze desiderate dei truster

T = B_pinv*tau;

% Conversione delle forze desiderate dei truster in numero di giri
b1 = 0.0003883;
u = T/b1;
offset = 31.5;   %limite della zona morta
n = zeros(7,1);
for i = 1:1:7
    n(i) = sign(u(i))*sqrt(abs(u(i)));
    n(i) = n(i) + sign(n(i))*offset;
end
n_des = n;

== matlab function mixTest123/Mission Supervisor/Trasf. in NED ==
  data: posArg input; pos output; areaOfInterestCorner parameter
function pos = LLD2NED(posArg,areaOfInterestCorner)
    coder.extrinsic('evalin','wgs84Ellipsoid','geodetic2ned');
    pos = zeros(1,3);
    pos1 = 0;
    pos2 = 0;
    pos3 = 0;
    [pos1, pos2, pos3] = geodetic2ned(posArg(1), posArg(2), posArg(3),areaOfInterestCorner(1), areaOfInterestCorner(2), 0,wgs84Ellipsoid);
    pos = [pos1, pos2, posArg(3)];
end

== matlab function mixTest123/controller/compute_if_enable ==
  settings: updateMethod=DISCRETE  sampleTime=0.1
  data: current_state input size=[8 1]; enable output size=[6 1]
function enable = fcn(current_state)
enable = zeros(6,1);
for i = 1:1:length(current_state)
    if (current_state(i) == 1 && i <= 5)
        enable(i) = 1;
    end
    if i > 5
        if (current_state(i) == 1 && i == 7)
            enable = zeros(6,1);
            enable(2) = 1;
        end
        if (current_state(i) == 1 && i == 8)
            enable = zeros(6,1);
            enable(2) = 0;
            enable(6) = 1;
        end
    end
end
end
